simulink model "Project6Simulink"  (R2020a)
settings: Solver=VariableStepAuto  StartTime=0.0  StopTime=Sim_time  RelTol=1e-3
values from neighbouring files (symbols this model uses):
  Cn = 2.3 * 3600    (= 8280)    [Project6.m]
  I = 2.3    [Project6.m]
  OCV = Data(:,2)    [Project6.m]
  R_charge = Data(:,3)    [Project6.m]
  R_discharge = Data(:,4)    [Project6.m]
  SOC = Data(:,1)    [Project6.m]
settings Model: Creator=cresp  LastModifiedBy=cresp

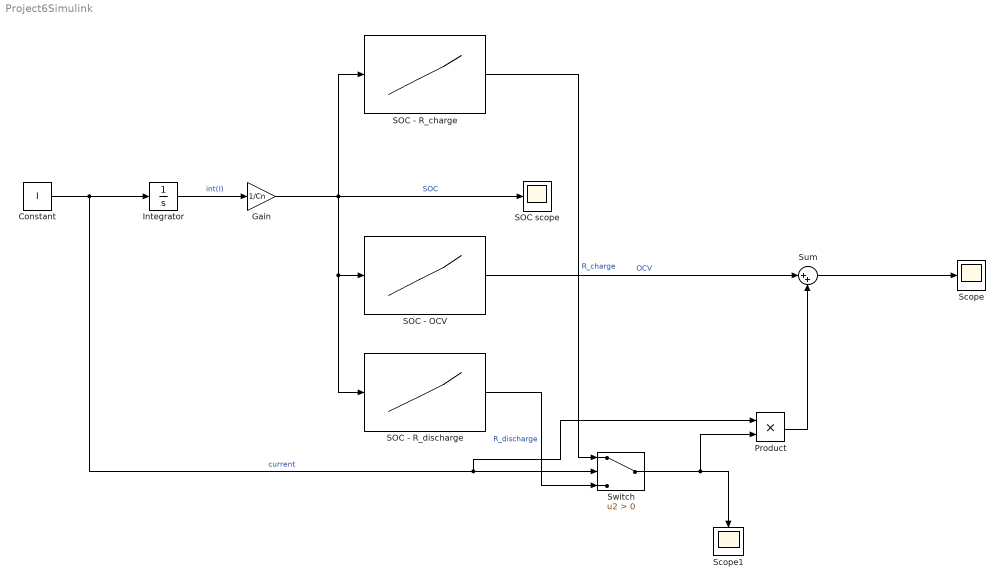
== system Project6Simulink ==
  Constant : Constant  Value=I
  Gain : Gain  Gain=1/Cn
  Integrator : Integrator
  Product : Product
  SOC - OCV : Lookup_n-D  NumberOfTableDimensions=1  BreakpointsForDimension1=SOC  Table=OCV  InternalRulePriority=Speed  RndMeth=Simplest  InputSameDT=on
  SOC - R_charge : Lookup_n-D  NumberOfTableDimensions=1  BreakpointsForDimension1=SOC  Table=R_charge  InternalRulePriority=Speed  RndMeth=Simplest  InputSameDT=on
  SOC - R_discharge : Lookup_n-D  NumberOfTableDimensions=1  BreakpointsForDimension1=SOC  Table=R_discharge  InternalRulePriority=Speed  RndMeth=Simplest  InputSameDT=on
  SOC scope : Scope
  Scope : Scope
  Scope1 : Scope
  Sum : Sum  Inputs=|++
  Switch : Switch  Criteria=u2 > Threshold
  wires:
  Constant/1 -> Product/1, Switch/2, Integrator/1  "current"
  Integrator/1 -> Gain/1  "int(I)"
  Gain/1 -> SOC - R_charge/1, SOC scope/1, SOC - R_discharge/1, SOC - OCV/1  "SOC"
  SOC - OCV/1 -> Sum/1  "OCV"
  SOC - R_discharge/1 -> Switch/3  "R_discharge"
  SOC - R_charge/1 -> Switch/1  "R_charge"
  Sum/1 -> Scope/1
  Switch/1 -> Scope1/1, Product/2
  Product/1 -> Sum/2
